simulink model "minjerk"  (R2023b)
settings: Solver=VariableStepAuto  StartTime=0.0  StopTime=10.0  RelTol=1e-3
values from neighbouring files (symbols this model uses):
  joint_angle = qrt(2:end,:)    [load_robot.m]
  joint_time = qrt(1,:)    [load_robot.m]
libraries: shareduavrstlib x1
settings Model: Creator=hp  LastModifiedBy=hp

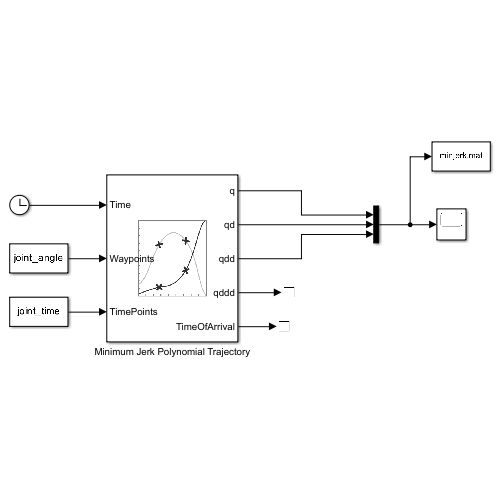
[thumbnail: Simulink's stored preview of the top-level diagram]
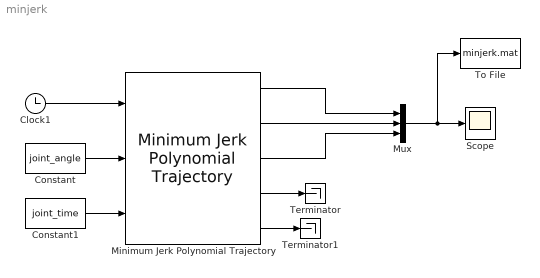
== system minjerk ==
  Clock1 : Clock
  Constant : Constant  Value=joint_angle
  Constant1 : Constant  Value=joint_time
  Minimum Jerk Polynomial Trajectory : shareduavrstlib/Minimum Jerk Polynomial Trajectory  ShowBCInputPort=off  ShowPolynomialCoefs=off  ShowStatusOutputPort=off  TimeAllocation=off  TimeWeight=100  MinSegmentTime=0.1  MaxSegmentTime=1  MaxIteration=1500  MaxTime=10  SimulateUsing=Interpreted execution
      settings: LibrarySourceBlock=robotutilslib/Minimum Jerk Polynomial Trajectory
  Mux : Mux  Inputs=3
  Scope : Scope
  Terminator : Terminator
  Terminator1 : Terminator
  To File : ToFile  Filename=minjerk.mat  MatrixName=minjerk  SampleTime=0.001
  wires:
  Clock1/1 -> Minimum Jerk Polynomial Trajectory/1
  Constant1/1 -> Minimum Jerk Polynomial Trajectory/3
  Constant/1 -> Minimum Jerk Polynomial Trajectory/2
  Minimum Jerk Polynomial Trajectory/4 -> Terminator/1
  Minimum Jerk Polynomial Trajectory/5 -> Terminator1/1
  Minimum Jerk Polynomial Trajectory/1 -> Mux/1
  Minimum Jerk Polynomial Trajectory/2 -> Mux/2
  Minimum Jerk Polynomial Trajectory/3 -> Mux/3
  Mux/1 -> To File/1, Scope/1
